simulink model "tarefa9e10"  (R2022b)
settings: Solver=VariableStepAuto  StartTime=0.0  StopTime=30  RelTol=1e-3
values from neighbouring files (symbols this model uses):
  d = -0.15    [lab9e10.m]
  p1 = b1*q0    [lab9e10.m]
  P1 = Q0*b1    [lab9e10.m]
  p2 = b2*q0    [lab9e10.m]
  P2 = Q0*(b2 - b1) + b1/(b1+b2)    [lab9e10.m]
  P3 = b2*(-Q0 + 1/(b1+b2))    [lab9e10.m]
  q0 = 1/(b1+b2)    [lab9e10.m]
  Q0 = 0.8*q0    [lab9e10.m]
  q1 = a1*q0    [lab9e10.m]
  Q1 = Q0*(a1-1) + 1/(b1+b2)    [lab9e10.m]
  q2 = a2*q0    [lab9e10.m]
  Q2 = Q0*(a2-a1) + a1/(b1+b2)    [lab9e10.m]
  Q3 = a2*(-Q0 + 1/(b1+b2))    [lab9e10.m]
  R = 1.25    [lab9e10.m]
  T0 = 0.201    [lab9e10.m]
  td = 15    [lab9e10.m]
undefined symbols (not defined in the file or in its folder): Gden, Gnum
settings Model: Creator=hugo_  LastModifiedBy=hugo_

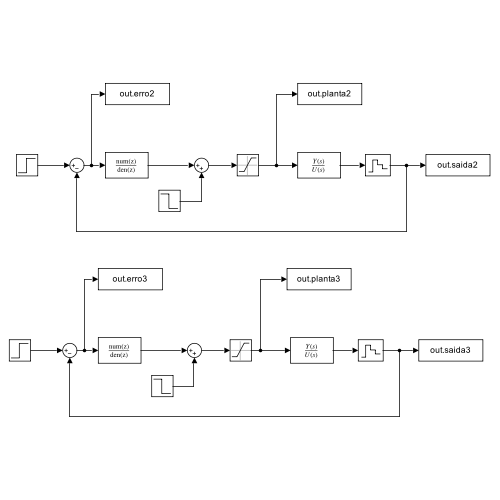
[thumbnail: Simulink's stored preview of the top-level diagram]
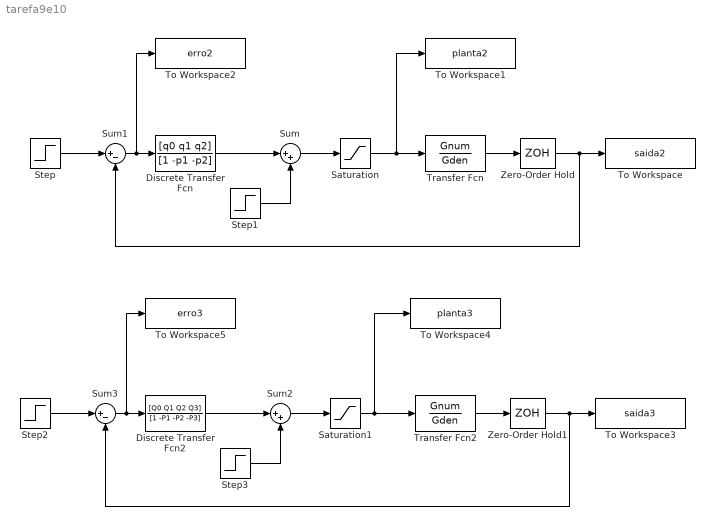
== system tarefa9e10 ==
  Discrete Transfer Fcn : DiscreteTransferFcn  Numerator=[q0 q1 q2]  Denominator=[1 -p1 -p2]  SampleTime=T0
  Discrete Transfer Fcn2 : DiscreteTransferFcn  Numerator=[Q0 Q1 Q2 Q3]  Denominator=[1 -P1 -P2 -P3]  SampleTime=T0
  Saturation : Saturate  UpperLimit=10  LowerLimit=-10
  Saturation1 : Saturate  UpperLimit=10  LowerLimit=-10
  Step : Step  Time=0  After=R  SampleTime=0
  Step1 : Step  Time=td  After=d  SampleTime=0
  Step2 : Step  Time=0  After=R  SampleTime=0
  Step3 : Step  Time=td  After=d  SampleTime=0
  Sum : Sum  Inputs=|++
  Sum1 : Sum  Inputs=|+-
  Sum2 : Sum  Inputs=|++
  Sum3 : Sum  Inputs=|+-
  To Workspace : ToWorkspace  VariableName=saida2  SaveFormat=Timeseries  SampleTime=-1
  To Workspace1 : ToWorkspace  VariableName=planta2  SaveFormat=Timeseries  SampleTime=-1
  To Workspace2 : ToWorkspace  VariableName=erro2  SaveFormat=Timeseries  SampleTime=-1
  To Workspace3 : ToWorkspace  VariableName=saida3  SaveFormat=Timeseries  SampleTime=-1
  To Workspace4 : ToWorkspace  VariableName=planta3  SaveFormat=Timeseries  SampleTime=-1
  To Workspace5 : ToWorkspace  VariableName=erro3  SaveFormat=Timeseries  SampleTime=-1
  Transfer Fcn : TransferFcn  Numerator=Gnum  Denominator=Gden
  Transfer Fcn2 : TransferFcn  Numerator=Gnum  Denominator=Gden
  Zero-Order Hold : ZeroOrderHold  SampleTime=-1
  Zero-Order Hold1 : ZeroOrderHold  SampleTime=-1
  wires:
  Discrete Transfer Fcn/1 -> Sum/1
  Sum1/1 -> To Workspace2/1, Discrete Transfer Fcn/1
  Transfer Fcn/1 -> Zero-Order Hold/1
  Sum/1 -> Saturation/1
  Saturation/1 -> Transfer Fcn/1, To Workspace1/1
  Step/1 -> Sum1/1
  Zero-Order Hold/1 -> To Workspace/1, Sum1/2
  Step1/1 -> Sum/2
  Step3/1 -> Sum2/2
  Sum2/1 -> Saturation1/1
  Sum3/1 -> To Workspace5/1, Discrete Transfer Fcn2/1
  Step2/1 -> Sum3/1
  Zero-Order Hold1/1 -> To Workspace3/1, Sum3/2
  Discrete Transfer Fcn2/1 -> Sum2/1
  Saturation1/1 -> Transfer Fcn2/1, To Workspace4/1
  Transfer Fcn2/1 -> Zero-Order Hold1/1
